simulink model "model_matematyczny_2018a1"  (R2018b)
settings: Solver=VariableStepAuto  StartTime=0.0  StopTime=30  RelTol=1e-3
libraries: powerlib_meascontrol x1
settings Model: Creator=Admin  LastModifiedBy=Student
settings DataIOCC: ReturnWorkspaceOutputs=on
settings DebuggingCC: UnconnectedInputMsg=none  UnconnectedOutputMsg=none  UnconnectedLineMsg=none  SFMachineParentedDataDiag=error

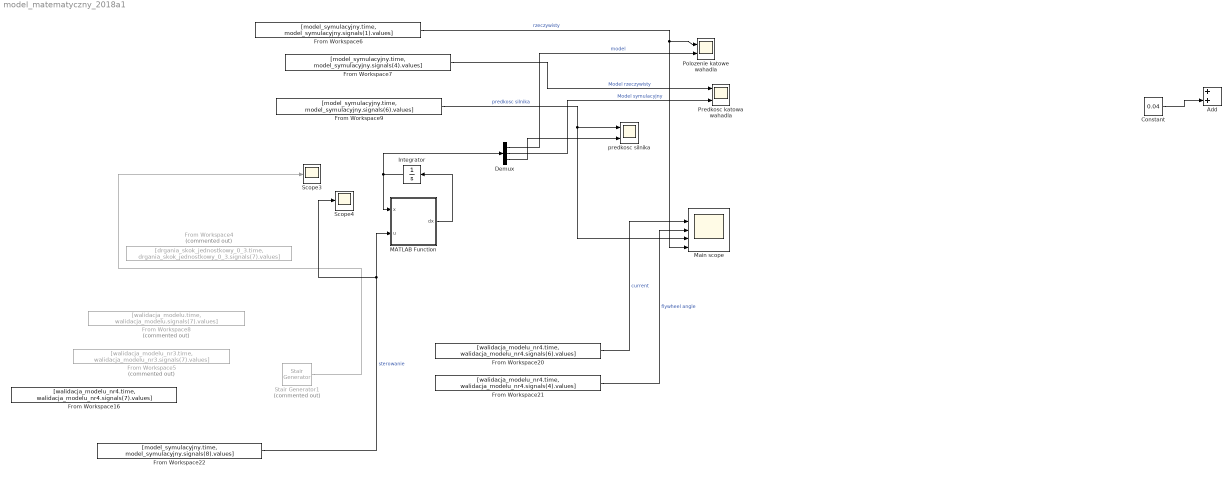
== system model_matematyczny_2018a1 ==
  Add : Sum
  Constant : Constant  Value=0.04
  Demux : Demux  Outputs=3
  From Workspace16 : FromWorkspace  VariableName=[walidacja_modelu_nr4.time, walidacja_modelu_nr4.signals(7).values]  SampleTime=0
  From Workspace20 : FromWorkspace  VariableName=[walidacja_modelu_nr4.time, walidacja_modelu_nr4.signals(6).values]  SampleTime=0
  From Workspace21 : FromWorkspace  VariableName=[walidacja_modelu_nr4.time, walidacja_modelu_nr4.signals(4).values]  SampleTime=0
  From Workspace22 : FromWorkspace  VariableName=[model_symulacyjny.time, model_symulacyjny.signals(8).values]  SampleTime=0
  From Workspace4 : FromWorkspace  Commented=on  VariableName=[drgania_skok_jednostkowy_0_3.time, drgania_skok_jednostkowy_0_3.signals(7).values]  SampleTime=0
  From Workspace5 : FromWorkspace  Commented=on  VariableName=[walidacja_modelu_nr3.time, walidacja_modelu_nr3.signals(7).values]  SampleTime=0
  From Workspace6 : FromWorkspace  VariableName=[model_symulacyjny.time, model_symulacyjny.signals(1).values]  SampleTime=0
  From Workspace7 : FromWorkspace  VariableName=[model_symulacyjny.time, model_symulacyjny.signals(4).values]  SampleTime=0
  From Workspace8 : FromWorkspace  Commented=on  VariableName=[walidacja_modelu.time, walidacja_modelu.signals(7).values]  SampleTime=0
  From Workspace9 : FromWorkspace  VariableName=[model_symulacyjny.time, model_symulacyjny.signals(6).values]  SampleTime=0
  Integrator : Integrator  InitialCondition=[0, 0, 0]
  MATLAB Function : MATLAB Function  TreatAsAtomicUnit=on
  "Main scope " : Scope  NumInputPorts=5
  "Polozenie katowe wahadla " : Scope  NumInputPorts=2
  "Predkosc katowa wahadla " : Scope  NumInputPorts=2
  Scope3 : Scope
  Scope4 : Scope
  Stair Generator1 : powerlib_meascontrol/Pulse & Signal Generators/Stair Generator  Commented=on  t=time  e=amp  Ts=0
      settings: SourceProductName=Simscape Power Systems
  "predkosc silnika " : Scope  NumInputPorts=2
  wires:
  MATLAB Function/1(dx) -> Integrator/1
  Integrator/1 -> MATLAB Function/1(x), Demux/1
  Demux/2 -> "Predkosc katowa wahadla "/2  "Model symulacyjny"
  Demux/3 -> "predkosc silnika "/2
  Demux/1 -> "Polozenie katowe wahadla "/2  "model"
  ? -> Add/1
  Constant/1 -> Add/2
  From Workspace6/1 -> "Main scope "/5, "Polozenie katowe wahadla "/1  "rzeczywisty"
  From Workspace7/1 -> "Predkosc katowa wahadla "/1  "Model rzeczywisty"
  Stair Generator1/1 -> Scope3/1
  From Workspace20/1 -> "Main scope "/2  "current"
  From Workspace9/1 -> "Main scope "/4, "predkosc silnika "/1  "predkosc silnika"
  From Workspace21/1 -> "Main scope "/3  "flywheel angle"
  From Workspace22/1 -> MATLAB Function/2(u), Scope4/1  "sterowanie"

== matlab function model_matematyczny_2018a1/MATLAB Function ==
  data: x input; u input; dx output
% function dx = fcn(x, u)
% 
% %dane wyidentyfikowane
% MgL = 0.1064;
% g = 9.81;
% kt = 0.027; % NmA
% R = 0.4; %Ohmy
% 
% mi_phi = 0.000082; 
% % mi_phi = 1.566850664740816e-04;
% % mi_theta = 0.0290; %zostało wyznaczone z drgań swobodnych 
% mi_theta = 0.0290;
% 
% G = 488.7;
% J = 0.0283; %kg*m^2
% 
% %wspołczynnik a:
% % a = 0.0023;
% % b = -0.0022;
% p = [0.002321260244060,-0.002210724041962];
% dx = [0 0 0];
% dx(1) = x(2); % pochodna polozenia
% dx(2) = (1/J)*(MgL * sin(x(1)) - mi_theta * x(2) + (((kt * kt)/R) + mi_phi) * x(3) - kt*u/R); % pochodna predkosci obrotowe belki
% dx(3) = G * (u - polyval(p, x(3))); %pochodna predkosci smigla 
% 
% end


function dx = fcn(x, u)

%dane wyidentyfikowane
MgL = 0.1264;
g = 9.81;
kt = 0.027; % NmA
ke = 0.025;
R = 2.4; %Ohmy

% mi_phi = 0.000644785835713765; 
mi_phi = 0.0000882;
% mi_theta = 0.00000132; %zostało wyznaczone z drgań swobodnych 
mi_theta = 0.0290;

G = 488.648;
% J = 0.0185; %kg*m^2
J = 0.0254;
%wspołczynnik a:
% a = 0.0023;
% b = -0.0022;
p = [0.002314296507890,-8.816367649105842e-04]
p_volt = [11.823766233766237,0.009523809523809];
dx = [0 0 0];
dx(1) = x(2); % pochodna polozenia
% dx(2) = (1/J)*(-MgL * sin(x(1)) - mi_theta * x(2) + (((kt * ke)/R) + mi_phi) * x(3) - kt*u/R); % pochodna predkosci obrotowe belki
dx(2) = (1/J)*(-MgL * sin(x(1)) - mi_theta * x(2) - (kt * (polyval(p_volt, u) - ke * x(3)) / R) + mi_phi * x(3));
dx(3) = G * (u - polyval(p, x(3))); %pochodna predkosci smigla 

end
